simulink model "SIMULINK_INVERSE_CONTROL_SANTIAGO_GARCIA"  (R2020a)
settings: Solver=FixedStepAuto  StartTime=0.0  StopTime=500  FixedStep=0.001  RelTol=1e-3
libraries: simulink x1
settings Model: Creator=USUARIO  LastModifiedBy=USUARIO

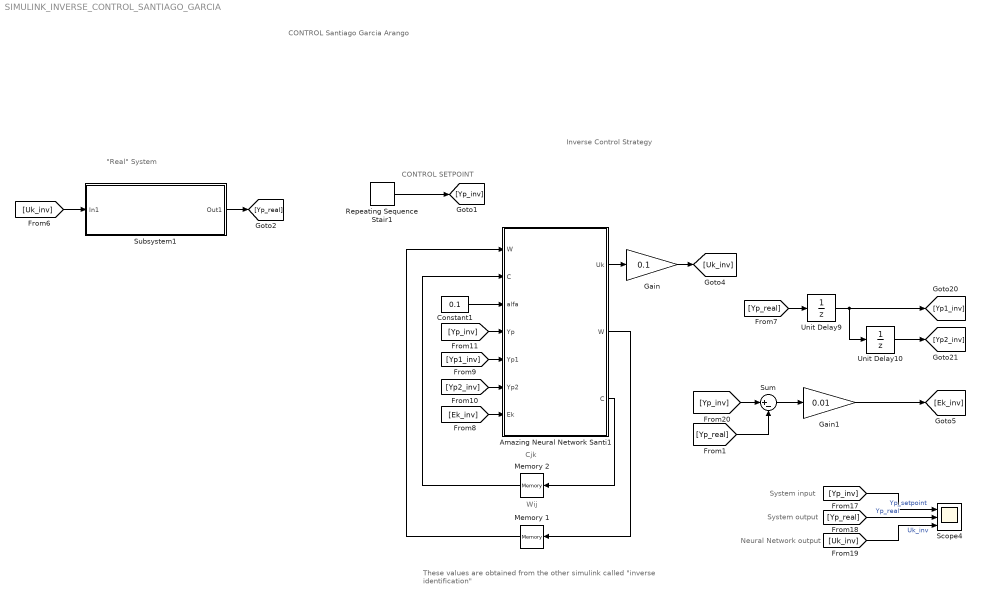
== system SIMULINK_INVERSE_CONTROL_SANTIAGO_GARCIA ==
  note: Inverse Control Strategy
  note: CONTROL SETPOINT
  note: System output
  note: System input
  note: Neural Network output
  note: "Real" System
  note: CONTROL
      | Santiago Garcia Arango
  note: Cjk
  note: Wij
  note: These values are obtained from the other simulink called
      | "inverse identification"
  " Memory 1" : Memory  InitialCondition=[-1.24800000000000,-0.145400000000000,1.09420000000000;-0.398800000000000,-0.0894000000000000,0.761600000000000;0.313100000000000,1.46030000000000,-0.332800000000000;3.60620000000000,1.43670000000000,0.321500000000000;2.72750000000000,1.37530000000000,-0.829000000000000;-1.36150000000000,0.659800000000000,0.876800000000000;3.02210000000000,-1.22030000000000,-1.15980000000000;0.748400000000000,0.740200000000000,-1.04590000000000;-0.0453000000000000,1.64790000000000,-0.791800000000000;0.682000000000000,0.456200000000000,-2.97690000000000]
  Amazing Neural Network Santi1 : MATLAB Function  TreatAsAtomicUnit=on
  Constant1 : Constant  Value=0.1
  Gain : Gain  Gain=0.1
  Gain1 : Gain  Gain=0.01
  Memory 2 : Memory  InitialCondition=[1.35060000000000,0.372700000000000,-0.635900000000000,1.59060000000000,-1.53410000000000,-0.0596000000000000,-0.161300000000000,0.383200000000000,0.399600000000000,-0.995400000000000]
  Repeating Sequence Stair1 : simulink/Sources/Repeating Sequence Stair  OutValues=[0 0.2 0.2 0.3 0.4 0.3 0.2].'  tsamp=50  OutMin=[]  OutMax=[]  OutDataTypeStr=double  OutputDataTypeScalingMode=double  OutDataType=fixdt(0,8)  ConRadixGroup=Best Precision: Vector-wise  OutScaling=2^-12
  Scope4 : Scope  NumInputPorts=3
  Subsystem1 : Subsystem
  Sum : Sum  Inputs=|+-
  Unit Delay10 : UnitDelay  SampleTime=-1  HasFrameUpgradeWarning=on
  Unit Delay9 : UnitDelay  SampleTime=-1  HasFrameUpgradeWarning=on
  wires:
  Repeating Sequence Stair1/1 -> [Yp_inv]
  [Yp_real] -> Sum/2
  [Yp_real] -> Scope4/2  "Yp_real"
  Sum/1 -> Gain1/1
  [Yp_inv] -> Scope4/1  "Yp_setpoint"
  Unit Delay10/1 -> [Yp2_inv]
  [Uk_inv] -> Scope4/3  "Uk_inv"
  [Yp_real] -> Unit Delay9/1
  Unit Delay9/1 -> [Yp1_inv], Unit Delay10/1
  [Yp_inv] -> Sum/1
  Subsystem1/1(Out1) -> [Yp_real]
  [Uk_inv] -> Subsystem1/1(In1)
  Amazing Neural Network Santi1/3(C) -> Memory 2/1
  Constant1/1 -> Amazing Neural Network Santi1/3(alfa)
  Amazing Neural Network Santi1/2(W) -> " Memory 1"/1
  Memory 2/1 -> Amazing Neural Network Santi1/2("C ")
  [Ek_inv] -> Amazing Neural Network Santi1/7(Ek)
  [Yp1_inv] -> Amazing Neural Network Santi1/5(Yp1)
  " Memory 1"/1 -> Amazing Neural Network Santi1/1("W ")
  [Yp_inv] -> Amazing Neural Network Santi1/4(Yp)
  [Yp2_inv] -> Amazing Neural Network Santi1/6(Yp2)
  Amazing Neural Network Santi1/1(Uk) -> Gain/1
  Gain/1 -> [Uk_inv]
  Gain1/1 -> [Ek_inv]

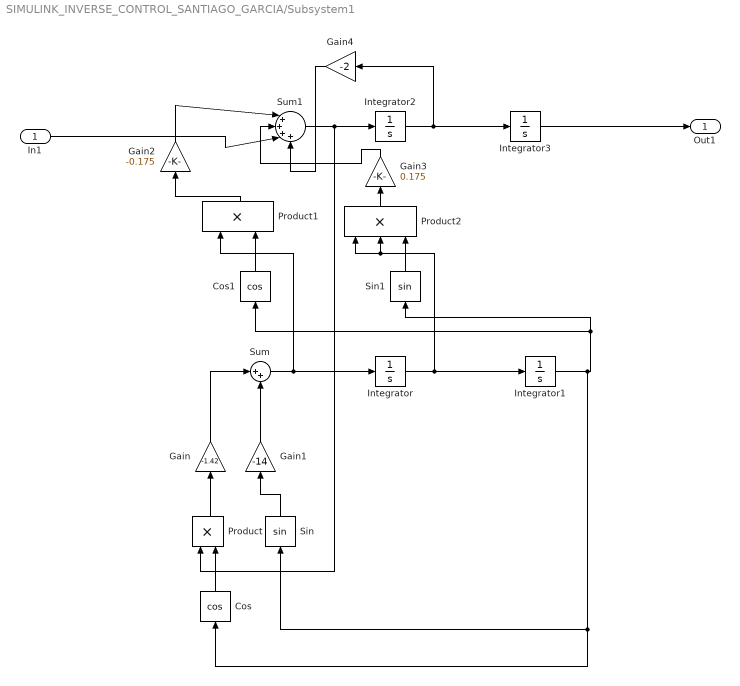
== system SIMULINK_INVERSE_CONTROL_SANTIAGO_GARCIA/Subsystem1 ==
  In1 : Inport
  Cos : Trigonometry  Operator=cos
  Cos1 : Trigonometry  Operator=cos
  Gain : Gain  Gain=-1.42
  Gain1 : Gain  Gain=-14
  Gain2 : Gain  Gain=-0.175
  Gain3 : Gain  Gain=0.175
  Gain4 : Gain  Gain=-2
  Integrator{,1..3} (4 alike) : Integrator
  Product : Product
  Product1 : Product
  Product2 : Product  Inputs=3
  Sin : Trigonometry
  Sin1 : Trigonometry
  Sum : Sum  Inputs=|++
  Sum1 : Sum  Inputs=|++++
  Out1 : Outport  VectorParamsAs1DForOutWhenUnconnected=off
  wires:
  Cos1/1 -> Product1/2
  Gain/1 -> Sum/1
  Product1/1 -> Gain2/1
  Sin1/1 -> Product2/3
  Gain1/1 -> Sum/2
  Gain3/1 -> Sum1/2
  Product/1 -> Gain/1
  Gain2/1 -> Sum1/1
  Sin/1 -> Gain1/1
  Cos/1 -> Product/2
  Sum1/1 -> Product/1, Integrator2/1
  Integrator2/1 -> Gain4/1, Integrator3/1
  In1/1 -> Sum1/3
  Integrator1/1 -> Sin/1, Cos/1, Cos1/1, Sin1/1
  Integrator3/1 -> Out1/1
  Gain4/1 -> Sum1/4
  Integrator/1 -> Integrator1/1, Product2/1, Product2/2
  Sum/1 -> Integrator/1, Product1/1
  Product2/1 -> Gain3/1

== matlab function SIMULINK_INVERSE_CONTROL_SANTIAGO_GARCIA/Amazing Neural Network Santi1 ==
  data: W input; Uk output; C input; alfa input; Yp input; Yp1 input; Yp2 input; W output; C output; Ek input
% NEURAL NETWORK FOR SIMULINK "REAL-TIME" PROCESSING BASED ON SIGNALS
% Santiago Garcia Arango
% ------------------------------------------------------------------------
% FEEDFORWARDMADALINE. Train or Test a simple neural network.
%   alfa: Learning rate constant (1 x 1)
%   W: vector of the initial Weights. size (1 x ne)
%   C: matrix of the initial hidden layers weights. size (ns x no+1)
%   REMARK: This processing is based on an "Inverse Identification"
% ------------------------------------------------------------------------

function [Uk, W, C] = fcn(W, C, alfa, Yp, Yp1, Yp2, Ek)

activation_function_1 = "tanh";
activation_function_2 = "none";

X = [Yp Yp1 Yp2]; % Create "entries" vector
Aj = W*X'; % Add hidden layer

if (activation_function_1 == "tanh")
    H = tanh(Aj);
end

Ak = C'*H; % Add output layer

if (activation_function_2 == "none")
    Uk = Ak;
end

C = C+alfa*Ek*H; % Update weights of C

if (activation_function_1 == "tanh")
    H2 = sech(H).^2;
end

W = W+alfa*Ek*(C.*H2)*X; % Update weights of W

end
